simulink model "calosc"  (R2018b)
settings: Solver=ode4  StartTime=0.0  StopTime=10.0  FixedStep=0.01  RelTol=1e-3
settings Model: Creator=User  LastModifiedBy=User
settings SolverCC: AlgebraicLoopSolver=LineSearch

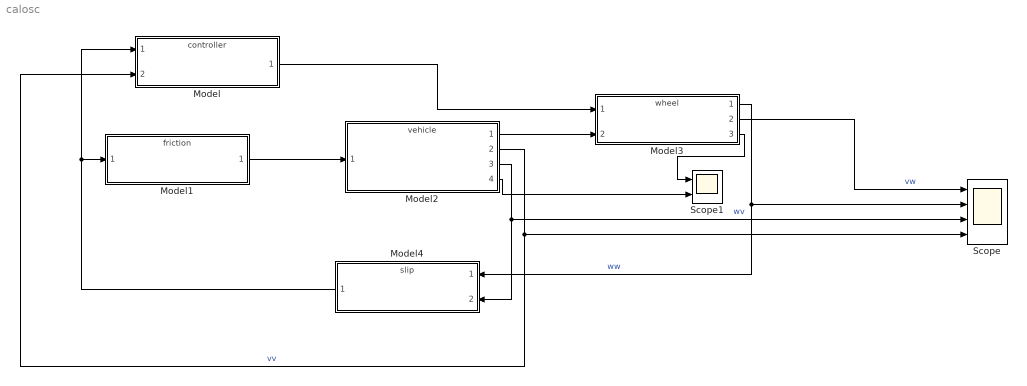
== system calosc ==
  Model : ModelReference  ModelNameDialog=controller.slx  SimulationMode=Normal  ModelReferenceVersion=1.2
  Model1 : ModelReference  ModelNameDialog=friction.slx  SimulationMode=Normal  ModelReferenceVersion=1.6
  Model2 : ModelReference  ModelNameDialog=vehicle.slx  SimulationMode=Normal  ModelReferenceVersion=1.2
  Model3 : ModelReference  ModelNameDialog=wheel.slx  SimulationMode=Normal  ModelReferenceVersion=1.2
  Model4 : ModelReference  ModelNameDialog=slip.slx  SimulationMode=Normal  ModelReferenceVersion=1.2
  Scope : Scope  NumInputPorts=4
  Scope1 : Scope  NumInputPorts=2
  wires:
  Model1/1 -> Model2/1
  Model2/1 -> Model3/2
  Model/1 -> Model3/1
  Model3/1 -> Scope/2, Model4/1  "ww"
  Model4/1 -> Model/1, Model1/1
  Model2/2 -> Model/2, Scope/4  "vv"
  Model3/2 -> Scope/1  "vw"
  Model3/3 -> Scope1/1
  Model2/4 -> Scope1/2
  Model2/3 -> Scope/3, Model4/2  "wv"
